simulink model "CorsoSimulink_1"  (R2019b)
settings: Solver=FixedStepAuto  StartTime=0.0  StopTime=10.0  FixedStep=0.001  RelTol=1e-3  EnableMultiTasking=on
settings Model: PacingRate=0.710000  Creator=SIMONE  LastModifiedBy=SIMONE
settings SolverCC: AutoInsertRateTranBlk=on
settings OptimizationCC: DefaultParameterBehavior=Inlined  UseDivisionForNetSlopeComputation=on  GainParamInheritBuiltInType=on  UseFloatMulNetSlope=on  InlineInvariantSignals=on  PassReuseOutputArgsAs=Individual arguments  ZeroExternalMemoryAtStartup=off  ZeroInternalMemoryAtStartup=off  NoFixptDivByZeroProtection=on  EfficientFloat2IntCast=on  LifeSpan=1  OptimizeBlockOrder=speed  DifferentSizesBufferReuse=on  EfficientTunableParamExpr=on
settings DebuggingCC: ParameterTunabilityLossMsg=error
settings HardwareCC: ProdBitPerPointer=32  ProdBitPerSizeT=32  ProdBitPerPtrDiffT=32  ProdLargestAtomicInteger=Long  ProdLargestAtomicFloat=Double  ProdWordSize=32  ProdLongLongMode=on  ProdHWDeviceType=ARM Compatible->ARM Cortex
settings SFSimCC: MATLABDynamicMemAlloc=off
settings RTWCC: SystemTargetFile=ert.tlc  TemplateMakefile=ert_default_tmf  GenerateReport=on  IncludeHyperlinkInReport=on  LaunchReport=on  GenerateTraceInfo=on  GenerateTraceReport=on  GenerateTraceReportSl=on  GenerateTraceReportSf=on  GenerateTraceReportEml=on  GenerateCodeMetricsReport=on
settings CodeAppCC: ForceParamTrailComments=on  IgnoreCustomStorageClasses=off  OperatorAnnotations=on  SimulinkDataObjDesc=on  SFDataObjDesc=on  CustomSymbolStrGlobalVar=rt$N$M  CustomSymbolStrType=$N$M  CustomSymbolStrFcn=$N$M$F  CustomSymbolStrMacro=$N$M  InsertBlockDesc=on
settings ERTTargetCC: TargetLangStandard=C99 (ISO)  GenerateSampleERTMain=on  IncludeMdlTerminateFcn=off  CombineSignalStateStructs=on  SupportAbsoluteTime=off  SupportComplex=off  SupportNonInlinedSFcns=on  InlinedParameterPlacement=NonHierarchical  ERTCustomFileTemplate=example_file_process.tlc  ERTFilePackagingFormat=CompactWithDataFile

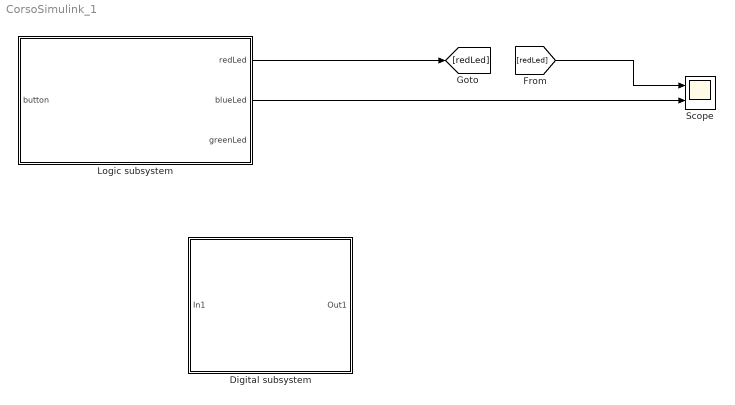
== system CorsoSimulink_1 ==
  Digital subsystem : Subsystem  TreatAsAtomicUnit=on  ScheduleAs=Periodic partition  PartitionName=Digital_subsystem  SystemSampleTime=0.001
  Logic subsystem : Subsystem  TreatAsAtomicUnit=on  ScheduleAs=Periodic partition  PartitionName=Logic_subsystem  SystemSampleTime=0.001
  Scope : Scope  NumInputPorts=2
  wires:
  Logic subsystem/1(redLed) -> [redLed]
  Logic subsystem/2(blueLed) -> Scope/2
  [redLed] -> Scope/1

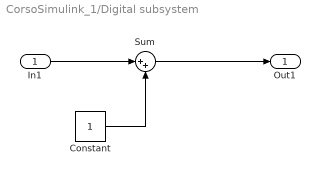
== system CorsoSimulink_1/Digital subsystem ==
  In1 : Inport
  Constant : Constant
  Sum : Sum  Inputs=|++
  Out1 : Outport
  wires:
  Constant/1 -> Sum/2
  In1/1 -> Sum/1
  Sum/1 -> Out1/1

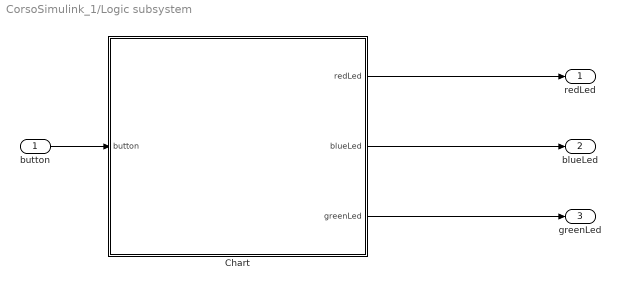
== system CorsoSimulink_1/Logic subsystem ==
  button : Inport
  Chart : Stateflow chart  BlockKeywords=__PRM__SERIALIZED__DATA__:Stateflow Chart,Stateflow Diagram  TreatAsAtomicUnit=on
  redLed : Outport
  blueLed : Outport  Port=2
  greenLed : Outport  Port=3
  wires:
  Chart/1(redLed) -> redLed/1
  Chart/2(blueLed) -> blueLed/1
  Chart/3(greenLed) -> greenLed/1
  button/1 -> Chart/1(button)

== stateflow chart CorsoSimulink_1/Logic subsystem/Chart ==
  state ACTIVE
    state BLUE_RED [parallel]
      settings: executionOrder=1
      state RED_ON
        entry:
        counter=0;
        redLed=1;
        during:
        counter++;
      state BLUE_ON
        entry:
        counter=0;
        blueLed=1;
        during:
        counter++;
      state RED_OFF
        entry:
        counter=0;
        redLed=0;
        during:
        counter++;
      state BLUE_OFF
        entry:
        counter=0;
        blueLed=0;
        during:
        counter++;
      (default) -> RED_ON
      RED_ON -> BLUE_ON : [counter>500]
      BLUE_ON -> RED_OFF : [counter>500]
      BLUE_OFF -> RED_ON : [counter>500]
      RED_OFF -> BLUE_OFF : [counter>500]
    state GREEN [parallel]
      settings: executionOrder=2
      state OFF
        en:
        counterGreen=0;
        greenLed=0;
        du:
        counterGreen++;
      state ON
        en:
        counterGreen=0;
        greenLed=1;
        du:
        counterGreen++;
      (default) -> ON
      ON -> OFF : [counterGreen>500]
      OFF -> ON : [counterGreen>500]
  state WAIT
    en:
    greenLed=0;
    blueLed=0;
    redLed=0;
  (default) -> ACTIVE
  ACTIVE -> WAIT : [button==1]
  WAIT -> ACTIVE : [button==1]
  data: counter local double size=1 =0; counterGreen local double size=1 =0; redLed output uint16 size=1 =uint16(0); blueLed output uint16 size=1 =uint16(0); greenLed output uint16 size=1 =uint16(0); button input double size=1
